simulink library "Pressure_Drop_StoragePipe"  (R2016b)
settings: Solver=ode45  StartTime=0.0  StopTime=10.0  RelTol=1e-3  EnableMultiTasking=on
libraries: carnot x2
settings Model: Creator=drhf  LastModifiedBy=drhf
settings DataIOCC: LimitDataPoints=on  SaveFormat=Array  SignalLoggingSaveFormat=ModelDataLogs
settings OptimizationCC: ExpressionDepthLimit=2147483647  LifeSpan=inf
settings DebuggingCC: UnderspecifiedInitializationDetection=Classic  MergeDetectMultiDrivingBlocksExec=none  SolverPrmCheckMsg=warning  FcnCallInpInsideContextMsg=warning  StateNameClashWarn=warning  SFUnexpectedBacktrackingDiag=warning  SFNoUnconditionalDefaultTransitionDiag=warning  SFExecutionAtInitializationDiag=none
settings HardwareCC: ProdBitPerPointer=32  ProdBitPerSizeT=32  ProdBitPerPtrDiffT=32  ProdLargestAtomicFloat=None  ProdIntDivRoundTo=Undefined  ProdEndianess=Unspecified  ProdWordSize=32  ProdHWDeviceType=32-bit Generic
settings ModelReferenceCC: PropagateSignalLabelsOutOfModel=off
settings GRTTargetCC: TargetLangStandard=C89/C90 (ANSI)  GeneratePreprocessorConditionals=Disable all  CombineOutputUpdateFcns=off  GRTInterface=on
settings ConfigComp: CovMetricSettings=dw  CovHtmlReporting=on  CovSaveCumulativeToWorkspaceVar=on  CovSaveSingleToWorkspaceVar=on  CovExternalEMLEnable=off

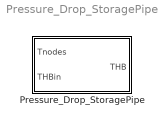
== system Pressure_Drop_StoragePipe ==
  Pressure_Drop_StoragePipe : Subsystem  mask(Pressure drop pipe connection of a storage){dia=0.03, hgt=1}
      mask prompts: dia "Diameter of pipe in m"; hgt "Height difference inlet-outlet"
      mask help: Calculates the pressure drop in a pipe connection to a storage respecting the diameter changes and the static height difference. The temperature for the density is taken from the storage nodes.
      mask Help: web(fullfile(path_carnot('help'),'Pressure_Drop_StoragePipe.html'),'-helpbrowser')
      mask TypeOptions dia: Pressure_Drop_changeD/dia
      mask TypeOptions hgt: Constant/Value

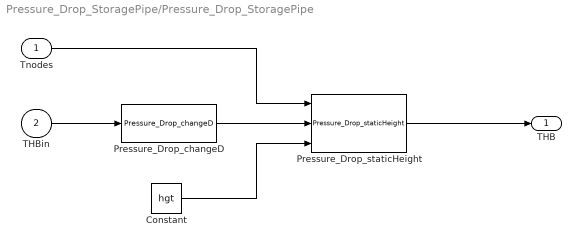
== system Pressure_Drop_StoragePipe/Pressure_Drop_StoragePipe ==
  Tnodes : Inport
  THBin : Inport  Port=2
  Constant : Constant  Value=hgt
  Pressure_Drop_changeD : carnot/Basic/Pressure_Drop/Pressure_Drop_changeD  dia=dia
  Pressure_Drop_staticHeight : carnot/Basic/Pressure_Drop/Pressure_Drop_staticHeight
  THB : Outport
  wires:
  Pressure_Drop_staticHeight/1 -> THB/1
  Tnodes/1 -> Pressure_Drop_staticHeight/1
  Pressure_Drop_changeD/1 -> Pressure_Drop_staticHeight/2
  Constant/1 -> Pressure_Drop_staticHeight/3
  THBin/1 -> Pressure_Drop_changeD/1
